simulink model "dllModel"  (R2018b)
settings: Solver=FixedStepDiscrete  StartTime=0.0  StopTime=10  FixedStep=0.1  RelTol=1e-3  EnableMultiTasking=on
undefined symbols (not defined in the file or in its folder): K, K2
settings Model: SimulationMode=accelerator  Creator=C3038028  LastModifiedBy=user
settings DataIOCC: SaveOutput=off  SignalLogging=off  VisualizeSimOutput=off  SaveTime=off
settings OptimizationCC: BlockReduction=off  ConditionallyExecuteInputs=off  DefaultParameterBehavior=Inlined  DefaultUnderspecifiedDataType=single  LifeSpan=Inf
settings DebuggingCC: AllowSymbolicDim=off  SFUnexpectedBacktrackingDiag=warning  SFNoUnconditionalDefaultTransitionDiag=warning  SFExecutionAtInitializationDiag=none
settings HardwareCC: TargetBitPerPointer=64  TargetBitPerSizeT=64  TargetBitPerPtrDiffT=64  TargetLongLongMode=on  TargetIntDivRoundTo=Zero  TargetEndianess=LittleEndian  TargetWordSize=64  TargetHWDeviceType=MATLAB Host  ProdEqTarget=off
settings ModelReferenceCC: PropagateSignalLabelsOutOfModel=off
settings SFSimCC: SimUseLocalCustomCode=off  MATLABDynamicMemAlloc=off
settings RTWCC: SystemTargetFile=ert_shrlib.tlc  TemplateMakefile=ert_default_tmf  Description=Embedded Coder (host-based shared library target)  RTWUseLocalCustomCode=off  BuildConfiguration=Faster Runs
settings CodeAppCC: IgnoreCustomStorageClasses=off  StateflowObjectComments=on
settings STFCustomTargetCC: GenerateSampleERTMain=on  ParMdlRefBuildCompliant=on  CompOptLevelCompliant=on  CombineOutputUpdateFcns=on  ERTCustomFileBanners=on  SupportContinuousTime=off  SupportNonInlinedSFcns=off  RemoveResetFunc=on  MATLABClassNameForMDSCustomization=Simulink.SoftwareTarget.ERTCustomization  ModelStepFunctionPrototypeControlCompliant=on  UseToolchainInfoCompliant=on  SystemTargetFile=ert_shrlib.tlc
settings ERTTargetCC: MultiwordLength=2048  GenerateSampleERTMain=on  ConcurrentExecutionCompliant=off  CPPClassGenCompliant=off  InlinedParameterPlacement=NonHierarchical  ERTCustomFileTemplate=example_file_process.tlc  ConvertIfToSwitch=off  SuppressUnreachableDefaultCases=off
settings ConfigComp: CovMetricSettings=dw  CovHtmlReporting=on  CovSaveCumulativeToWorkspaceVar=on  CovSaveSingleToWorkspaceVar=on  CovExternalEMLEnable=off

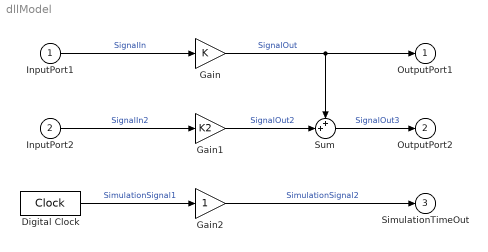
== system dllModel ==
  InputPort1 : Inport  OutDataTypeStr=single
  InputPort2 : Inport  Port=2  OutDataTypeStr=uint16
  Digital Clock : DigitalClock  SampleTime=0.1
  Gain : Gain  Gain=K  OutDataTypeStr=single
  Gain1 : Gain  Gain=K2  OutDataTypeStr=uint16
  Gain2 : Gain  OutDataTypeStr=Inherit: Same as input
  Sum : Sum  Inputs=++|
  OutputPort1 : Outport
  OutputPort2 : Outport  Port=2
  SimulationTimeOut : Outport  Port=3
  wires:
  InputPort1/1 -> Gain/1  "SignalIn"
  Gain/1 -> OutputPort1/1, Sum/1  "SignalOut"
  InputPort2/1 -> Gain1/1  "SignalIn2"
  Sum/1 -> OutputPort2/1  "SignalOut3"
  Gain1/1 -> Sum/2  "SignalOut2"
  Gain2/1 -> SimulationTimeOut/1  "SimulationSignal2"
  Digital Clock/1 -> Gain2/1  "SimulationSignal1"
